simulink model "wheeled_pendulum_linear_ADRC"  (R2018b)
settings: Solver=VariableStepAuto  StartTime=0.0  StopTime=30  RelTol=1e-3
InitFcn:
  | %%%%%%%%%%%%%%%%%%%%%%%%%
  | %                     TUNABLE PARAMETERS                 %
  | %    (ORDER, SETTLING TIME, ESO GAIN AND B0)  %
  | %%%%%%%%%%%%%%%%%%%%%%%%%
  | order = 3;                     % ADRC order
  | ts = 5;                        % Desired settling time
  | b0 = 0.5;                         % b0 parameter
  | eso_gain = 15;                % ESO Dynamic related to closed-loop poles
  | 
  | %%%%%%%%%%%%%%%%%%%%%%%%%
  | %                                 ADRC                               %
  | %      (CONTROLLER GAINS AND ESO MATRIXES)    %
  | %%%%%%%%%%%%%%%%%%%%%%%%%
  | s_cl = 4/ts;                           % Closed-loop system poles
  | s_eso = eso_gain * s_cl;        % ESO poles
  | pole = [1 s_cl];                     % Base polynomial to calculate
  |                                            % System characteristic polynomial
  | pole_eso = [1 s_eso];            % Base polynomial to calculate
  |                                            % ESO characteristic polynomial
  | A = zeros(order + 1);            % Matrix A of ESO
  | B = zeros(order + 1, 1);        % Matrix B of ESO
  | C = [1 zeros(1, order)];         % Matrix C of ESO
  | 
  | %%%%%%%%%%%%%%%%%%%%%%%%%%%%%%%%%%%
  | % Here we'll calculate the characteristic polynomials of system and ESO,   %
  | % starting with the base polynomial, and convoluting it until we achieve    %
  | % the system's order.                                                                           %
  | % Also, we'll put the values of A and B matrixes of ESO, filling the             %
  | % diagonal above the main diagonal of A with one's, and putting the value %
  | % b0 on the penultimate value of B matrix, according to ADRC generalized %
  | % model fot Nth order.                                                                          %
  | %%%%%%%%%%%%%%%%%%%%%%%%%%%%%%%%%%%
  | A_sys = pole;
  | A_eso = pole_eso;
  | 
  | for i = 1:order
  |     if i ~= order
  |         A_sys = conv(A_sys, pole);
  |     else
  |         B(i) = b0;
  |     end
  |     A(i,i+1) = 1;
  |     A_eso = conv(A_eso, pole_eso);
  | end
  | 
  | K = [1 A_sys(2:end)];           % Controller gain matrix
  | L = A_eso(2:end)';               % ESO gain matrix
  | 
  | %%%%%%%%%%%%%%%%%%%%%%%%%
  | %                    SYSTEM PARAMETERS              %
  | %%%%%%%%%%%%%%%%%%%%%%%%%
  | r = 3.15e-2;           % wheel radius
  | mw = 3.15e-2;       % wheel mass
  | l = 8.36e-3;            % distance between COG and wheel axle
  | mb = 0.3604;         % inner body mass
  | d = 0.177;              % wheels distance
  | ja = 8.1367e-5;      % inner body moment of inertia about wheel axle A
  | jb = 5.74620e-4;    % inner body moment of inertia about axis B
  | k = 64;                   % gear ratio
  | jr = 0.12e-7;           % rotor inertia
  | R = 2.3;                  % rotor resistance
  | L = 2.6e-5;             % rotor inductance
  | km = 2.05e-3;        % torque
  | ke = 2.05e-3;         % Back-EMF
  | b = 2.1e-5;             % body-motor viscous friction coefficient
  | fv = 1.8e-4;            % wheels-ground viscous friction coefficient
  | g = 9.81;                % gravity
  | 
  | Tf_aux = [b + fv, 0, -b;
  |           0, b + fv, -b;
  |          -b, -b, 2 * b];
  | 
  | Ta_aux = km * k * [1, 0;
  |                    0, 1;
  |                   -1, -1];
  | 
  | I_aux = ke * k * [1, 0, -1;
  |                   0, 1, -1];
  | 
  | K_aux = ((l^2 * r^2) / d^2) * mb;
undefined symbols (not defined in the file): AM, Am, ffth, frst, frth, O, scnd, t1, t2, t3, t4, thrd, TM, Tm
libraries: dspindex x2, dspmtrx3 x1
settings Model: Creator=root  LastModifiedBy=root

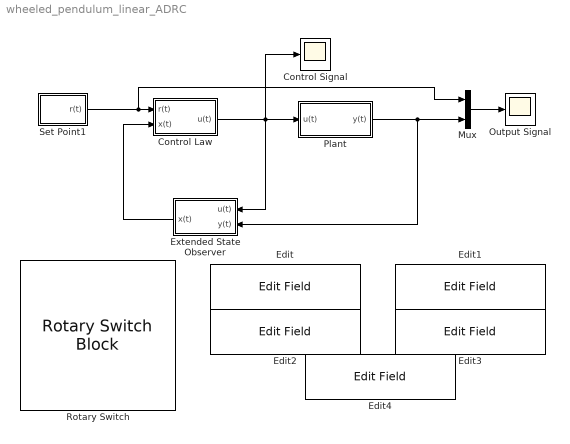
== system wheeled_pendulum_linear_ADRC ==
  Control Law : Subsystem
  Control Signal : Scope
  Edit : EditField  WebBlockId=108  ShowInitialText=on  Alignment=Center
  Edit1 : EditField  WebBlockId=109  ShowInitialText=on  Alignment=Center
  Edit2 : EditField  WebBlockId=110  ShowInitialText=on  Alignment=Center
  Edit3 : EditField  WebBlockId=111  ShowInitialText=on  Alignment=Center
  Edit4 : EditField  WebBlockId=112  ShowInitialText=on  Alignment=Center
  Extended State Observer : Subsystem
  Mux : Mux  Inputs=2
  Output Signal : Scope
  Plant : Subsystem
  Rotary Switch : RotarySwitchBlock  WebBlockId=114
      settings: Values={{'Step', 'Sine', 'Sawtooth', 'Square', 'Random'}, [0 1 2 3 4]}
  Set Point1 : Subsystem
  wires:
  Plant/1(y(t)) -> Extended State Observer/2(y(t)), Mux/2
  Extended State Observer/1(x(t)) -> Control Law/2(x(t))
  Control Law/1(u(t)) -> Control Signal/1, Plant/1(u(t)), Extended State Observer/1("u(t) ")
  Set Point1/1(r(t)) -> Mux/1, Control Law/1(r(t))
  Mux/1 -> Output Signal/1

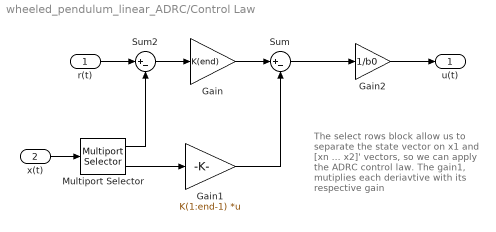
== system wheeled_pendulum_linear_ADRC/Control Law ==
  note: The select rows block allow us to separate the state vector on x1 and [xn ... x2]' vectors, so we can apply the ADRC control law. The gain1, mutiplies each deriavtive with its respective gain
  r(t) : Inport
  x(t) : Inport  Port=2
  Gain : Gain  Gain=K(end)  ParamDataTypeStr=Inherit: Inherit from 'Gain'
  Gain1 : Gain  Gain=K(1:end-1)  Multiplication=Matrix(K*u) (u vector)
  Gain2 : Gain  Gain=1/b0
  Multiport Selector : dspindex/Multiport Selector  rowsOrCols=Rows  idxCellArray={ 1, [order+1:-1:2]}  idxErrMode=Clip Index
  Sum : Sum  Inputs=|+-
  Sum2 : Sum  Inputs=|+-
  u(t) : Outport
  wires:
  Gain2/1 -> u(t)/1
  Sum/1 -> Gain2/1
  r(t)/1 -> Sum2/1
  Sum2/1 -> Gain/1
  Gain/1 -> Sum/1
  x(t)/1 -> Multiport Selector/1
  Multiport Selector/1 -> Sum2/2
  Multiport Selector/2 -> Gain1/1
  Gain1/1 -> Sum/2

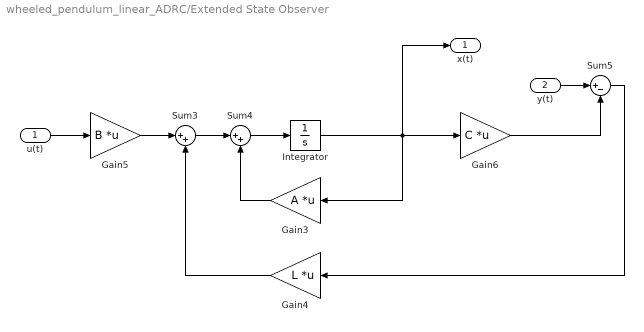
== system wheeled_pendulum_linear_ADRC/Extended State Observer ==
  "u(t) " : Inport
  y(t) : Inport  Port=2
  Gain3 : Gain  Gain=A  Multiplication=Matrix(K*u) (u vector)
  Gain4 : Gain  Gain=L  Multiplication=Matrix(K*u) (u vector)
  Gain5 : Gain  Gain=B  Multiplication=Matrix(K*u) (u vector)
  Gain6 : Gain  Gain=C  Multiplication=Matrix(K*u) (u vector)
  Integrator : Integrator
  Sum3 : Sum  Inputs=|++
  Sum4 : Sum  Inputs=|++
  Sum5 : Sum  Inputs=|+-
  x(t) : Outport
  wires:
  Sum4/1 -> Integrator/1
  y(t)/1 -> Sum5/1
  Gain4/1 -> Sum3/2
  Gain5/1 -> Sum3/1
  Gain3/1 -> Sum4/2
  Sum3/1 -> Sum4/1
  Sum5/1 -> Gain4/1
  Gain6/1 -> Sum5/2
  Integrator/1 -> x(t)/1, Gain3/1, Gain6/1
  "u(t) "/1 -> Gain5/1

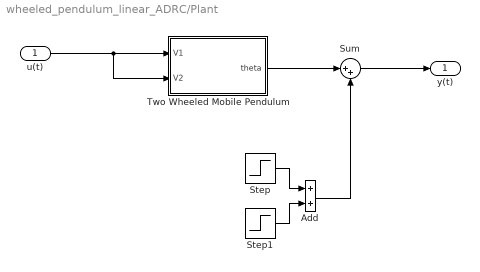
== system wheeled_pendulum_linear_ADRC/Plant ==
  u(t) : Inport
  Add : Sum
  Step : Step  Time=15  After=0.4  SampleTime=0
  Step1 : Step  Time=16  After=-0.4  SampleTime=0
  Sum : Sum  Inputs=|++
  Two Wheeled Mobile Pendulum : Subsystem
  y(t) : Outport
  wires:
  u(t)/1 -> Two Wheeled Mobile Pendulum/2(V2), Two Wheeled Mobile Pendulum/1(V1)
  Two Wheeled Mobile Pendulum/1(theta) -> Sum/1
  Sum/1 -> y(t)/1
  Step/1 -> Add/1
  Step1/1 -> Add/2
  Add/1 -> Sum/2

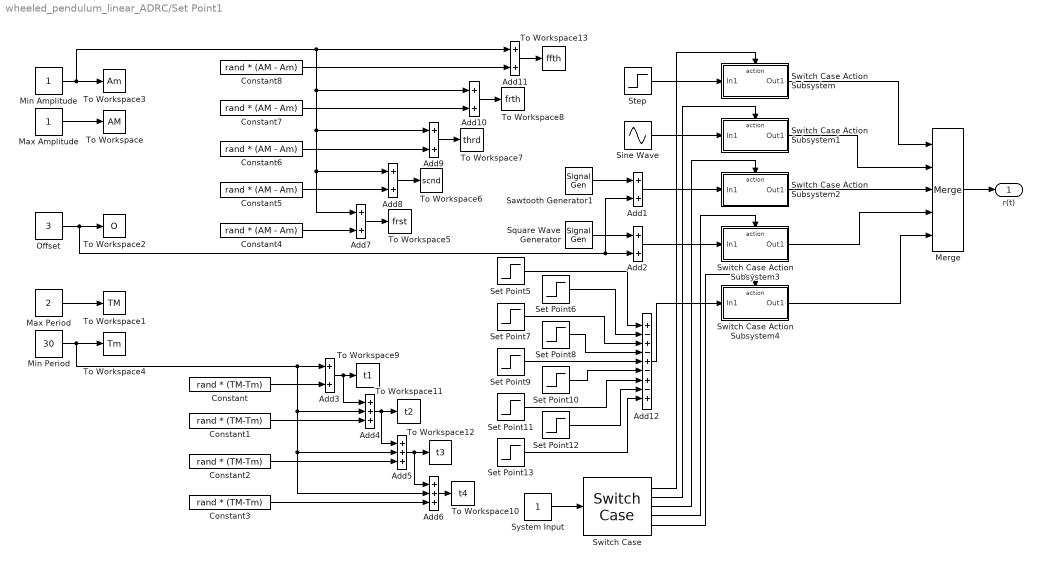
== system wheeled_pendulum_linear_ADRC/Set Point1 ==
  Add{1..3,7} (4 alike) : Sum  Inputs=2
  Add{8..11} (4 alike) : Sum
  Add12 : Sum  Inputs=+-+-+-+-+
  Add4 : Sum  Inputs=3
  Add5 : Sum  Inputs=3
  Add6 : Sum  Inputs=3
  Constant{,1..3} (4 alike) : Constant  Value=rand * (TM-Tm)
  Constant{4..8} (5 alike) : Constant  Value=rand * (AM - Am)
  Max Amplitude : Constant  VectorParams1D=off
  Max Period : Constant  Value=2  VectorParams1D=off
  Merge : Merge  Inputs=5
  Min Amplitude : Constant  VectorParams1D=off
  Min Period : Constant  Value=30  VectorParams1D=off
  Offset : Constant  Value=3  VectorParams1D=off
  Sawtooth Generator1 : SignalGenerator  WaveForm=sawtooth  Amplitude=AM  Frequency=1/TM  Units=rad/sec
  Set Point10 : Step  Time=t3  After=thrd  SampleTime=0
  Set Point11 : Step  Time=t3  After=frth  SampleTime=0
  Set Point12 : Step  Time=t4  After=frth  SampleTime=0
  Set Point13 : Step  Time=t4  After=ffth  SampleTime=0
  Set Point5 : Step  Time=0  After=frst  SampleTime=0
  Set Point6 : Step  Time=t1  After=frst  SampleTime=0
  Set Point7 : Step  Time=t1  After=scnd  SampleTime=0
  Set Point8 : Step  Time=t2  After=scnd  SampleTime=0
  Set Point9 : Step  Time=t2  After=thrd  SampleTime=0
  Sine Wave : Sin  Amplitude=AM  Bias=O  Frequency=1/TM  SampleTime=0
  Square Wave Generator : SignalGenerator  WaveForm=square  Amplitude=AM  Frequency=1/TM  Units=rad/sec
  Step : Step  Time=0  After=AM  SampleTime=0
  Switch Case : SwitchCase  CaseConditions={0,1,2,3,4}  ShowDefaultCase=off
  Switch Case Action Subsystem : Subsystem  TreatAsAtomicUnit=on
  Switch Case Action Subsystem1 : Subsystem  TreatAsAtomicUnit=on
  Switch Case Action Subsystem2 : Subsystem  TreatAsAtomicUnit=on
  Switch Case Action Subsystem3 : Subsystem  TreatAsAtomicUnit=on
  Switch Case Action Subsystem4 : Subsystem  TreatAsAtomicUnit=on
  System Input : Constant
  To Workspace : ToWorkspace  VariableName=AM  SampleTime=-1
      settings: MaxDataPoints=1
  To Workspace1 : ToWorkspace  VariableName=TM  SampleTime=-1
      settings: MaxDataPoints=1
  To Workspace10 : ToWorkspace  VariableName=t4  SampleTime=-1
      settings: MaxDataPoints=1
  To Workspace11 : ToWorkspace  VariableName=t2  SampleTime=-1
      settings: MaxDataPoints=1
  To Workspace12 : ToWorkspace  VariableName=t3  SampleTime=-1
      settings: MaxDataPoints=1
  To Workspace13 : ToWorkspace  VariableName=ffth  SampleTime=-1
      settings: MaxDataPoints=1
  To Workspace2 : ToWorkspace  VariableName=O  SampleTime=-1
      settings: MaxDataPoints=1
  To Workspace3 : ToWorkspace  VariableName=Am  SampleTime=-1
      settings: MaxDataPoints=1
  To Workspace4 : ToWorkspace  VariableName=Tm  SampleTime=-1
      settings: MaxDataPoints=1
  To Workspace5 : ToWorkspace  VariableName=frst  SampleTime=-1
      settings: MaxDataPoints=1
  To Workspace6 : ToWorkspace  VariableName=scnd  SampleTime=-1
      settings: MaxDataPoints=1
  To Workspace7 : ToWorkspace  VariableName=thrd  SampleTime=-1
      settings: MaxDataPoints=1
  To Workspace8 : ToWorkspace  VariableName=frth  SampleTime=-1
      settings: MaxDataPoints=1
  To Workspace9 : ToWorkspace  VariableName=t1  SampleTime=-1
      settings: MaxDataPoints=1
  r(t) : Outport
  wires:
  Merge/1 -> r(t)/1
  Switch Case Action Subsystem3/1(Out1) -> Merge/4
  Switch Case/1 -> Switch Case Action Subsystem/Action
  Max Amplitude/1 -> To Workspace/1
  Square Wave Generator/1 -> Add2/1
  Add1/1 -> Switch Case Action Subsystem2/1(In1)
  Step/1 -> Switch Case Action Subsystem/1(In1)
  Switch Case/3 -> Switch Case Action Subsystem2/Action
  Switch Case/4 -> Switch Case Action Subsystem3/Action
  Switch Case/5 -> Switch Case Action Subsystem4/Action
  Switch Case/2 -> Switch Case Action Subsystem1/Action
  Sawtooth Generator1/1 -> Add1/1
  System Input/1 -> Switch Case/1
  Switch Case Action Subsystem/1(Out1) -> Merge/1
  Add2/1 -> Switch Case Action Subsystem3/1(In1)
  Min Amplitude/1 -> To Workspace3/1, Add7/1, Add8/1, Add9/1, Add10/1, Add11/1
  Max Period/1 -> To Workspace1/1
  Offset/1 -> Add1/2, Add2/2, To Workspace2/1
  Switch Case Action Subsystem4/1(Out1) -> Merge/5
  Switch Case Action Subsystem2/1(Out1) -> Merge/3
  Sine Wave/1 -> Switch Case Action Subsystem1/1(In1)
  Switch Case Action Subsystem1/1(Out1) -> Merge/2
  Min Period/1 -> To Workspace4/1, Add6/2, Add5/2, Add4/2, Add3/1
  Add12/1 -> Switch Case Action Subsystem4/1(In1)
  Constant/1 -> Add3/2
  Add3/1 -> Add4/1, To Workspace9/1
  Add4/1 -> Add5/1, To Workspace11/1
  Constant1/1 -> Add4/3
  Constant2/1 -> Add5/3
  Add6/1 -> To Workspace10/1
  Add5/1 -> Add6/1, To Workspace12/1
  Constant3/1 -> Add6/3
  Add8/1 -> To Workspace6/1
  Add10/1 -> To Workspace8/1
  Add9/1 -> To Workspace7/1
  Add7/1 -> To Workspace5/1
  Constant4/1 -> Add7/2
  Constant5/1 -> Add8/2
  Constant6/1 -> Add9/2
  Constant7/1 -> Add10/2
  Add11/1 -> To Workspace13/1
  Constant8/1 -> Add11/2
  Set Point13/1 -> Add12/9
  Set Point11/1 -> Add12/7
  Set Point9/1 -> Add12/5
  Set Point8/1 -> Add12/4
  Set Point5/1 -> Add12/1
  Set Point12/1 -> Add12/8
  Set Point7/1 -> Add12/3
  Set Point10/1 -> Add12/6
  Set Point6/1 -> Add12/2

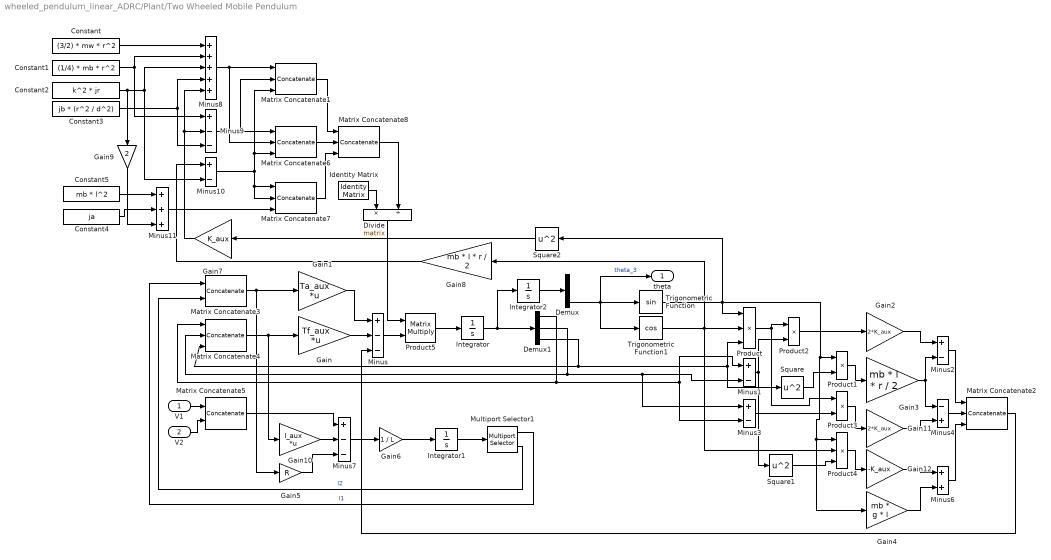
== system wheeled_pendulum_linear_ADRC/Plant/Two Wheeled Mobile Pendulum ==
  V1 : Inport
  V2 : Inport  Port=2
  Constant : Constant  Value=(3/2) * mw * r^2
  Constant1 : Constant  Value=(1/4) * mb * r^2
  Constant2 : Constant  Value=k^2 * jr
  Constant3 : Constant  Value=jb * (r^2 / d^2)
  Constant4 : Constant  Value=ja
  Constant5 : Constant  Value=mb * l^2
  Demux : Demux  Outputs=3
  Demux1 : Demux  Outputs=3
  Divide : Product  Inputs=*/  Multiplication=Matrix(*)
  Gain : Gain  Gain=Tf_aux  Multiplication=Matrix(K*u)
  Gain1 : Gain  Gain=Ta_aux  Multiplication=Matrix(K*u)
  Gain10 : Gain  Gain=I_aux  Multiplication=Matrix(K*u)
  Gain11 : Gain  Gain=2*K_aux
  Gain12 : Gain  Gain=-K_aux
  Gain2 : Gain  Gain=2*K_aux
  Gain3 : Gain  Gain=mb * l * r / 2
  Gain4 : Gain  Gain=mb * g * l
  Gain5 : Gain  Gain=R
  Gain6 : Gain  Gain=1 / L
  Gain7 : Gain  Gain=K_aux
  Gain8 : Gain  Gain=mb * l * r / 2
  Gain9 : Gain  Gain=2
  Identity Matrix : dspmtrx3/Identity Matrix  Inherit=off  N=3  Ts=1  dataType=double  isSigned=on  wordLen=16  udDataType=sfix(16)  fracBitsMode=Best precision  numFracBits=15  OutDataTypeStr=double  LastOutDataTypeStr=double
      settings: SourceProductName=DSP System Toolbox
  Integrator : Integrator
  Integrator1 : Integrator
  Integrator2 : Integrator
  Matrix Concatenate1 : Concatenate  NumInputs=3  Mode=Multidimensional array  ConcatenateDimension=2
  Matrix Concatenate2 : Concatenate  NumInputs=3  Mode=Multidimensional array
  Matrix Concatenate3 : Concatenate  Mode=Multidimensional array
  Matrix Concatenate4 : Concatenate  NumInputs=3  Mode=Multidimensional array
  Matrix Concatenate5 : Concatenate  Mode=Multidimensional array
  Matrix Concatenate6 : Concatenate  NumInputs=3  Mode=Multidimensional array  ConcatenateDimension=2
  Matrix Concatenate7 : Concatenate  NumInputs=3  Mode=Multidimensional array  ConcatenateDimension=2
  Matrix Concatenate8 : Concatenate  NumInputs=3  Mode=Multidimensional array
  Minus : Sum  Inputs=+--
  Minus{1..3,10} (4 alike) : Sum  Inputs=+-
  Minus11 : Sum  Inputs=+++
  Minus4 : Sum  Inputs=-+
  Minus6 : Sum
  Minus7 : Sum  Inputs=+--
  Minus8 : Sum  Inputs=+++++
  Minus9 : Sum  Inputs=+--
  Multiport Selector1 : dspindex/Multiport Selector  rowsOrCols=Rows  idxCellArray={1, 2}  idxErrMode=Clip Index
  Product : Product  Inputs=3
  Product1 : Product
  Product2 : Product
  Product3 : Product
  Product4 : Product  Inputs=3
  Product5 : Product  Multiplication=Matrix(*)
  Square : Math  Operator=square  SaturateOnIntegerOverflow=on
  Square1 : Math  Operator=square  SaturateOnIntegerOverflow=on
  Square2 : Math  Operator=square  SaturateOnIntegerOverflow=on
  Trigonometric Function : Trigonometry
  Trigonometric Function1 : Trigonometry  Operator=cos
  theta : Outport
  wires:
  Minus/1 -> Product5/2
  Product5/1 -> Integrator/1
  Matrix Concatenate8/1 -> Divide/2
  Constant5/1 -> Minus11/1
  Matrix Concatenate7/1 -> Matrix Concatenate8/3
  Multiport Selector1/1 -> Matrix Concatenate3/1  "I1"
  Square2/1 -> Gain7/1
  Matrix Concatenate4/1 -> Gain/1, Gain10/1
  Minus1/1 -> Product2/2, Square1/1
  Matrix Concatenate6/1 -> Matrix Concatenate8/2
  Minus4/1 -> Matrix Concatenate2/2
  Matrix Concatenate5/1 -> Minus7/1
  Gain2/1 -> Minus2/1
  Constant1/1 -> Minus8/2, Minus9/1
  Matrix Concatenate2/1 -> Minus/3
  Integrator2/1 -> Demux/1
  Trigonometric Function/1 -> Product4/1, Gain4/1, Product1/1, Product/1, Square2/1
  Product2/1 -> Gain2/1
  Demux/3 -> Trigonometric Function1/1, theta/1, Trigonometric Function/1  "theta_3"
  Minus3/1 -> Product3/2
  Trigonometric Function1/1 -> Product/2, Gain8/1, Product4/2
  Constant4/1 -> Minus11/2
  Product1/1 -> Gain3/1
  Minus10/1 -> Matrix Concatenate7/2, Matrix Concatenate7/1, Matrix Concatenate6/3, Matrix Concatenate1/3
  Gain7/1 -> Minus9/2, Minus8/5
  Integrator1/1 -> Multiport Selector1/1
  Divide/1 -> Product5/1
  Minus8/1 -> Matrix Concatenate6/2, Matrix Concatenate1/1
  Gain3/1 -> Minus4/1, Minus2/2
  V1/1 -> Matrix Concatenate5/1
  Demux1/3 -> Square/1, Product/3, Matrix Concatenate4/3
  Gain9/1 -> Minus11/3
  Product/1 -> Product2/1, Product3/1
  Gain4/1 -> Minus6/2
  Minus6/1 -> Matrix Concatenate2/3
  Minus9/1 -> Matrix Concatenate6/1, Matrix Concatenate1/2
  Gain1/1 -> Minus/1
  Gain6/1 -> Integrator1/1
  Product4/1 -> Gain12/1
  Constant/1 -> Minus8/1
  Demux1/1 -> Minus3/2, Minus1/1, Matrix Concatenate4/1
  V2/1 -> Matrix Concatenate5/2
  Identity Matrix/1 -> Divide/1
  Demux1/2 -> Minus1/2, Minus3/1, Matrix Concatenate4/2
  Matrix Concatenate3/1 -> Gain5/1, Gain1/1
  Gain10/1 -> Minus7/2
  Constant3/1 -> Minus8/4, Minus9/3
  Gain12/1 -> Minus6/1
  Square/1 -> Product1/2
  Gain11/1 -> Minus4/2
  Integrator/1 -> Demux1/1, Integrator2/1
  Constant2/1 -> Minus8/3, Minus10/2, Gain9/1
  Square1/1 -> Product4/3
  Minus11/1 -> Matrix Concatenate7/3
  Gain5/1 -> Minus7/3
  Matrix Concatenate1/1 -> Matrix Concatenate8/1
  Gain8/1 -> Minus10/1
  Product3/1 -> Gain11/1
  Gain/1 -> Minus/2
  Minus7/1 -> Gain6/1
  Minus2/1 -> Matrix Concatenate2/1
  Multiport Selector1/2 -> Matrix Concatenate3/2  "I2"

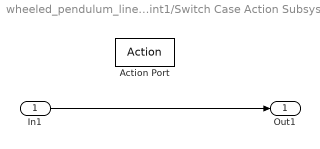
== system wheeled_pendulum_linear_ADRC/Set Point1/Switch Case Action Subsystem ==
  In1 : Inport
  Action Port : ActionPort
  Out1 : Outport
  wires:
  In1/1 -> Out1/1

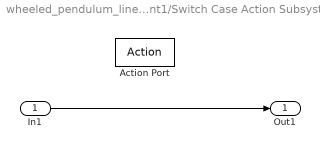
== system wheeled_pendulum_linear_ADRC/Set Point1/Switch Case Action Subsystem1 ==
  In1 : Inport
  Action Port : ActionPort
  Out1 : Outport
  wires:
  In1/1 -> Out1/1

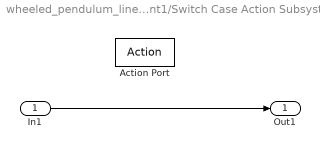
== system wheeled_pendulum_linear_ADRC/Set Point1/Switch Case Action Subsystem2 ==
  In1 : Inport
  Action Port : ActionPort
  Out1 : Outport
  wires:
  In1/1 -> Out1/1

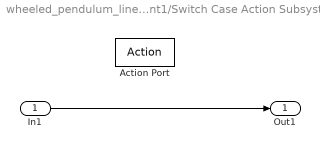
== system wheeled_pendulum_linear_ADRC/Set Point1/Switch Case Action Subsystem3 ==
  In1 : Inport
  Action Port : ActionPort
  Out1 : Outport
  wires:
  In1/1 -> Out1/1

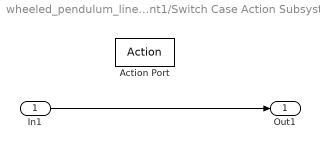
== system wheeled_pendulum_linear_ADRC/Set Point1/Switch Case Action Subsystem4 ==
  In1 : Inport
  Action Port : ActionPort
  Out1 : Outport
  wires:
  In1/1 -> Out1/1
